simulink model "ABC_model_Group_05"  (R2023a)
settings: Solver=VariableStepAuto  StartTime=0.0  StopTime=10.0  RelTol=1e-3
libraries: sharedutil x6, aerolibutil x2
settings Model: Creator=shivam  LastModifiedBy=shivam

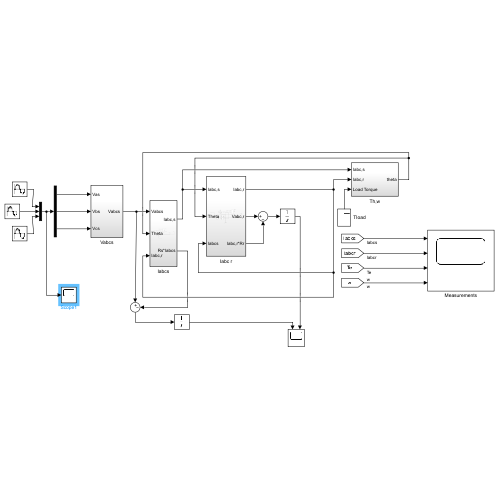
[thumbnail: Simulink's stored preview of the top-level diagram]
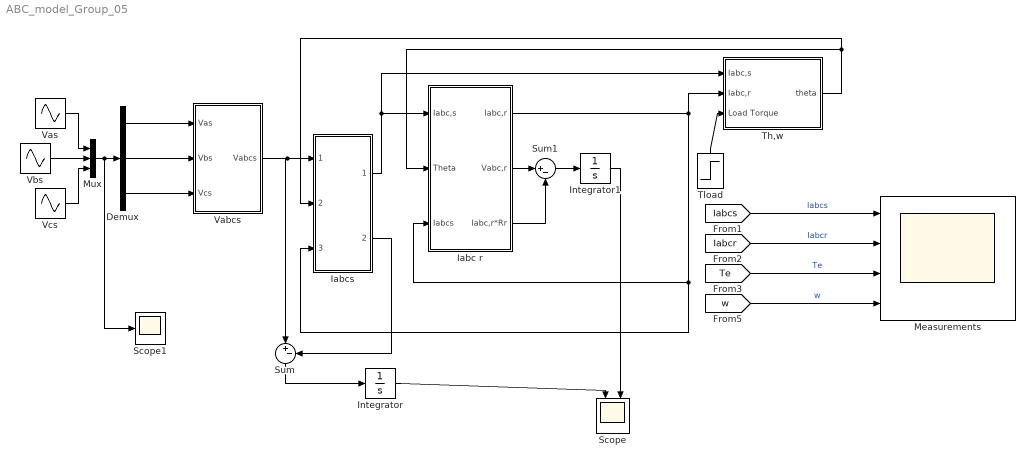
== system ABC_model_Group_05 ==
  Demux : Demux  Outputs=3
  Iabc r : Subsystem
  Iabcs : Subsystem
  Integrator : Integrator
  Integrator1 : Integrator
  "Measurements " : Scope  NumInputPorts=4
  Mux : Mux  Inputs=3
  Scope : Scope  NumInputPorts=2
  Scope1 : Scope
  Sum : Sum  Inputs=|+-
  Sum1 : Sum  Inputs=|+-
  Th,w : Subsystem
  Tload : Step  After=200.106  SampleTime=0
  Vabcs : Subsystem
  Vas : Sin  Amplitude=(460*sqrt(2))/sqrt(3)  Frequency=2*pi*60  Phase=(2*pi)/3  SampleTime=50e-6
  Vbs : Sin  Amplitude=(460*sqrt(2))/sqrt(3)  Frequency=2*pi*60  SampleTime=50e-6
  Vcs : Sin  Amplitude=(460*sqrt(2))/sqrt(3)  Frequency=2*pi*60  Phase=(4*pi)/3  SampleTime=50e-6
  wires:
  Vcs/1 -> Mux/3
  Vas/1 -> Mux/1
  Vbs/1 -> Mux/2
  Demux/3 -> Vabcs/3(Vcs)
  Demux/2 -> Vabcs/2(Vbs)
  Demux/1 -> Vabcs/1(Vas)
  Mux/1 -> Scope1/1, Demux/1
  Tload/1 -> Th,w/3(Load Torque)
  [w] -> "Measurements "/4  "w"
  [Te] -> "Measurements "/3  "Te"
  [Iabcr] -> "Measurements "/2  "Iabcr"
  [Iabcs] -> "Measurements "/1  "Iabcs"
  Vabcs/1("Vabcs ") -> Sum/1, Iabcs/1(Vabcs)
  Iabcs/2(Rs*Iabcs) -> Sum/2
  Sum/1 -> Integrator/1
  Integrator/1 -> Scope/1
  Th,w/1(theta) -> Iabcs/2(Theta), Iabc r/2(Theta)
  Iabcs/1(Iabc,s) -> Iabc r/1(Iabc,s), Th,w/1(Iabc,s)
  Iabc r/1(Iabc,r) -> Th,w/2(Iabc,r), Iabcs/3(Iabc,r), Iabc r/3(Iabcs)
  Iabc r/2(Vabc,r) -> Sum1/1
  Iabc r/3(Iabc,r*Rr) -> Sum1/2
  Sum1/1 -> Integrator1/1
  Integrator1/1 -> Scope/2

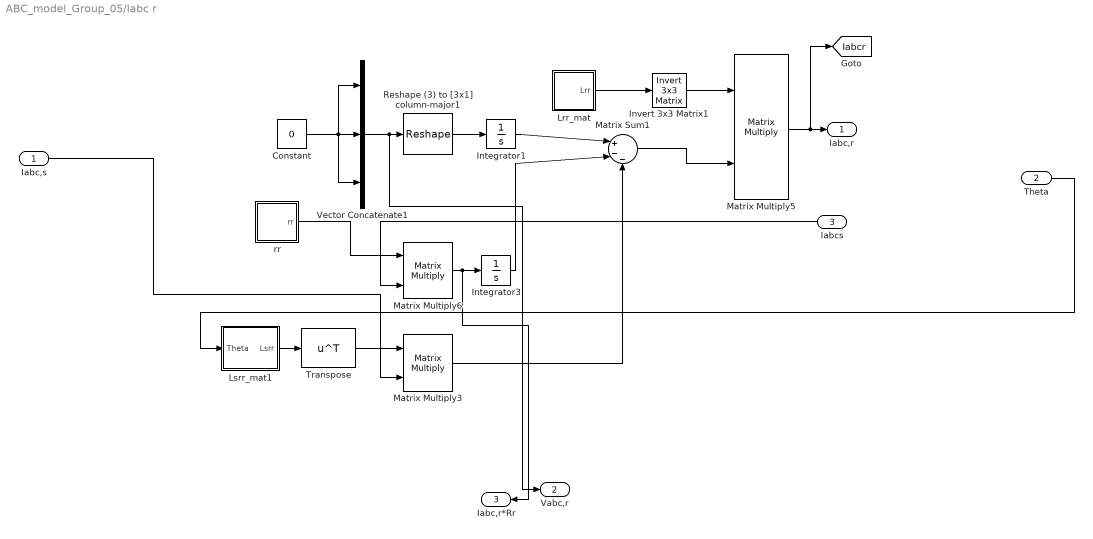
== system ABC_model_Group_05/Iabc r ==
  Iabc,s : Inport
  Theta : Inport  Port=2
  Iabcs : Inport  Port=3
  Constant : Constant  Value=0
  Integrator1 : Integrator
  Integrator3 : Integrator
  Invert 3x3 Matrix1 : aerolibutil/Invert  3x3 Matrix
  Lrr_mat : Subsystem
  Lsrr_mat1 : Subsystem
  Matrix Sum1 : Sum  Inputs=|+--
  Matrix Multiply3 : Product  Multiplication=Matrix(*)
  Matrix Multiply5 : Product  Multiplication=Matrix(*)
  Matrix Multiply6 : Product  Multiplication=Matrix(*)
  Reshape (3) to [3x1] column-major1 : Reshape  OutputDimensionality=Customize  OutputDimensions=[3,1]
  Transpose : Math  Operator=transpose
  Vector Concatenate1 : Concatenate  NumInputs=3
  rr : Subsystem
  Iabc,r : Outport
  Vabc,r : Outport  Port=2
  Iabc,r*Rr : Outport  Port=3
  tag scope: Iabcr=global
  wires:
  Matrix Multiply6/1 -> Iabc,r*Rr/1, Integrator3/1
  Integrator1/1 -> Matrix Sum1/1
  Theta/1 -> Lsrr_mat1/1(Theta)
  Iabc,s/1 -> Matrix Multiply3/2
  Constant/1 -> Vector Concatenate1/3, Vector Concatenate1/1, Vector Concatenate1/2
  Lrr_mat/1(Lrr) -> Invert 3x3 Matrix1/1
  Reshape (3) to [3x1] column-major1/1 -> Integrator1/1
  Vector Concatenate1/1 -> Vabc,r/1, Reshape (3) to [3x1] column-major1/1
  rr/1(rr) -> Matrix Multiply6/1
  Matrix Sum1/1 -> Matrix Multiply5/2
  Matrix Multiply3/1 -> Matrix Sum1/3
  Integrator3/1 -> Matrix Sum1/2
  Invert 3x3 Matrix1/1 -> Matrix Multiply5/1
  Matrix Multiply5/1 -> Iabc,r/1, [Iabcr]
  Iabcs/1 -> Matrix Multiply6/2
  Lsrr_mat1/1(Lsrr) -> Transpose/1
  Transpose/1 -> Matrix Multiply3/1

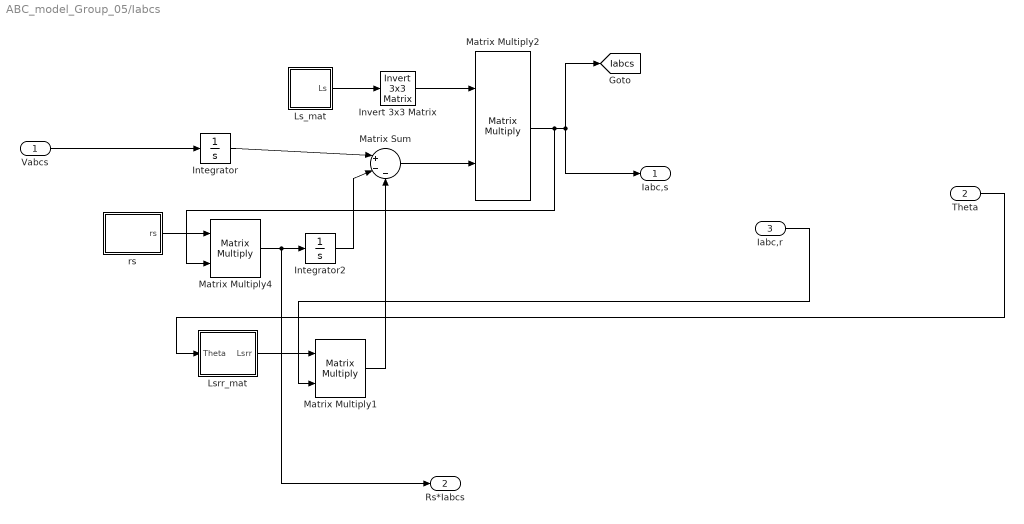
== system ABC_model_Group_05/Iabcs ==
  Vabcs : Inport
  Theta : Inport  Port=2
  Iabc,r : Inport  Port=3
  Integrator : Integrator
  Integrator2 : Integrator
  Invert 3x3 Matrix : aerolibutil/Invert  3x3 Matrix
  Ls_mat : Subsystem
  Lsrr_mat : Subsystem
  Matrix Sum : Sum  Inputs=|+--
  Matrix Multiply1 : Product  Multiplication=Matrix(*)
  Matrix Multiply2 : Product  Multiplication=Matrix(*)
  Matrix Multiply4 : Product  Multiplication=Matrix(*)
  rs : Subsystem
  Iabc,s : Outport
  Rs*Iabcs : Outport  Port=2
  tag scope: Iabcs=global
  wires:
  rs/1(rs) -> Matrix Multiply4/1
  Invert 3x3 Matrix/1 -> Matrix Multiply2/1
  Matrix Multiply4/1 -> Rs*Iabcs/1, Integrator2/1
  Vabcs/1 -> Integrator/1
  Ls_mat/1(Ls) -> Invert 3x3 Matrix/1
  Lsrr_mat/1(Lsrr) -> Matrix Multiply1/1
  Matrix Multiply2/1 -> Iabc,s/1, [Iabcs], Matrix Multiply4/2
  Matrix Multiply1/1 -> Matrix Sum/3
  Integrator2/1 -> Matrix Sum/2
  Matrix Sum/1 -> Matrix Multiply2/2
  Integrator/1 -> Matrix Sum/1
  Theta/1 -> Lsrr_mat/1(Theta)
  Iabc,r/1 -> Matrix Multiply1/2

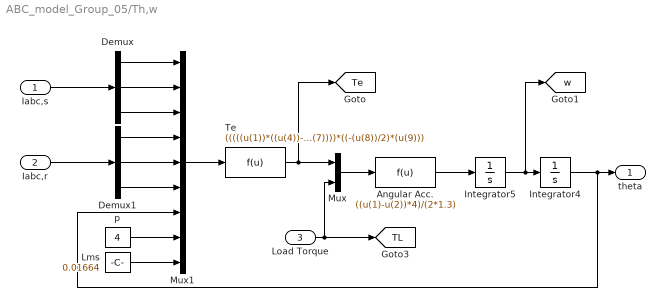
== system ABC_model_Group_05/Th,w ==
  Iabc,s : Inport
  Iabc,r : Inport  Port=2
  Load Torque : Inport  Port=3
  Angular Acc. : Fcn  Expr=((u(1)-u(2))*4)/(2*1.3)
  Demux : Demux  Outputs=3
  Demux1 : Demux  Outputs=3
  Integrator4 : Integrator
  Integrator5 : Integrator
  Lms : Constant  Value=0.01664
  Mux : Mux  Inputs=2
  Mux1 : Mux  Inputs=9
  Te : Fcn  Expr=(((((u(1))*((u(4))-(0.5*(u(5)))-(0.5*(u(6)))))+((u(2))*((u(5))-(0.5*(u(4)))-(0.5*(u(6)))))+((u(3))*((u(6))-(0.5*(u(5)))-(0.5*(u(4))))))*sin(u(7)))+((sqrt(3)/2)*(((u(1))*((u(5))-(u(6))))+((u(2))*((u(6))-(u(4))))+((u(3))*((u(4))-(u(5)))))*cos(u(7))))*((-(u(8))/2)*(u(9)))
  p : Constant  Value=4
  theta : Outport
  tag scope: TL=global, Te=global, w=global
  wires:
  Iabc,s/1 -> Demux/1
  Integrator4/1 -> Mux1/7, theta/1
  Mux/1 -> Angular Acc./1
  Load Torque/1 -> Mux/2, [TL]
  Angular Acc./1 -> Integrator5/1
  Te/1 -> [Te], Mux/1
  Integrator5/1 -> [w], Integrator4/1
  Iabc,r/1 -> Demux1/1
  Mux1/1 -> Te/1
  Demux/1 -> Mux1/1
  Demux/2 -> Mux1/2
  Demux/3 -> Mux1/3
  Demux1/1 -> Mux1/4
  Demux1/2 -> Mux1/5
  Demux1/3 -> Mux1/6
  p/1 -> Mux1/8
  Lms/1 -> Mux1/9

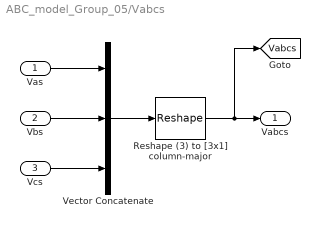
== system ABC_model_Group_05/Vabcs ==
  Vas : Inport
  Vbs : Inport  Port=2
  Vcs : Inport  Port=3
  Reshape (3) to [3x1] column-major : Reshape  OutputDimensionality=Customize  OutputDimensions=[3,1]
  Vector Concatenate : Concatenate  NumInputs=3
  "Vabcs " : Outport
  tag scope: Vabcs=global
  wires:
  Vector Concatenate/1 -> Reshape (3) to [3x1] column-major/1
  Reshape (3) to [3x1] column-major/1 -> [Vabcs], "Vabcs "/1
  Vbs/1 -> Vector Concatenate/2
  Vcs/1 -> Vector Concatenate/3
  Vas/1 -> Vector Concatenate/1

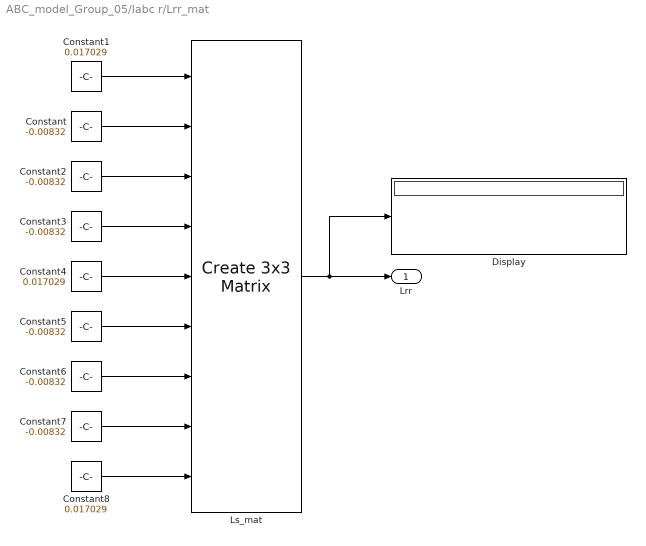
== system ABC_model_Group_05/Iabc r/Lrr_mat ==
  Constant{,2..3,5..7} (6 alike) : Constant  Value=-0.00832
  Constant1 : Constant  Value=0.017029
  Constant4 : Constant  Value=0.017029
  Constant8 : Constant  Value=0.017029
  Display : Display
  Ls_mat : sharedutil/Create 3x3 Matrix  aMode=aMode
      settings: LibrarySourceBlock=aerolibutil/Create 3x3 Matrix
  Lrr : Outport
  wires:
  Constant4/1 -> Ls_mat/5
  Constant5/1 -> Ls_mat/6
  Constant/1 -> Ls_mat/2
  Constant3/1 -> Ls_mat/4
  Constant1/1 -> Ls_mat/1
  Constant2/1 -> Ls_mat/3
  Constant6/1 -> Ls_mat/7
  Constant7/1 -> Ls_mat/8
  Constant8/1 -> Ls_mat/9
  Ls_mat/1 -> Display/1, Lrr/1

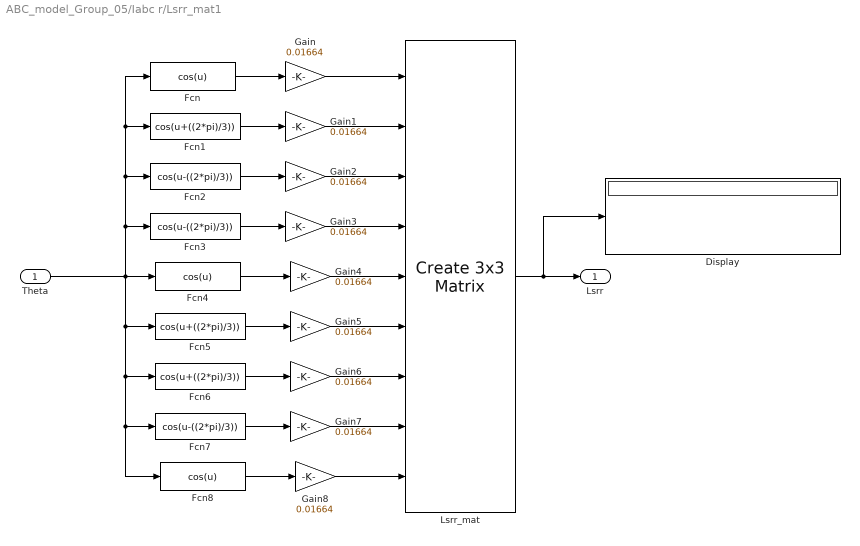
== system ABC_model_Group_05/Iabc r/Lsrr_mat1 ==
  Theta : Inport
  Display : Display
  Fcn : Fcn  Expr=cos(u)
  Fcn1 : Fcn  Expr=cos(u+((2*pi)/3))
  Fcn2 : Fcn  Expr=cos(u-((2*pi)/3))
  Fcn3 : Fcn  Expr=cos(u-((2*pi)/3))
  Fcn4 : Fcn  Expr=cos(u)
  Fcn5 : Fcn  Expr=cos(u+((2*pi)/3))
  Fcn6 : Fcn  Expr=cos(u+((2*pi)/3))
  Fcn7 : Fcn  Expr=cos(u-((2*pi)/3))
  Fcn8 : Fcn  Expr=cos(u)
  Gain{,1..8} (9 alike) : Gain  Gain=0.01664
  Lsrr_mat : sharedutil/Create 3x3 Matrix  aMode=aMode
      settings: LibrarySourceBlock=aerolibutil/Create 3x3 Matrix
  Lsrr : Outport
  wires:
  Fcn/1 -> Gain/1
  Fcn1/1 -> Gain1/1
  Fcn2/1 -> Gain2/1
  Gain/1 -> Lsrr_mat/1
  Gain1/1 -> Lsrr_mat/2
  Gain2/1 -> Lsrr_mat/3
  Fcn3/1 -> Gain3/1
  Gain3/1 -> Lsrr_mat/4
  Fcn4/1 -> Gain4/1
  Gain4/1 -> Lsrr_mat/5
  Fcn5/1 -> Gain5/1
  Gain5/1 -> Lsrr_mat/6
  Fcn6/1 -> Gain6/1
  Gain6/1 -> Lsrr_mat/7
  Fcn7/1 -> Gain7/1
  Gain7/1 -> Lsrr_mat/8
  Fcn8/1 -> Gain8/1
  Gain8/1 -> Lsrr_mat/9
  Theta/1 -> Fcn/1, Fcn1/1, Fcn2/1, Fcn3/1, Fcn5/1, Fcn6/1, Fcn8/1, Fcn7/1, Fcn4/1
  Lsrr_mat/1 -> Display/1, Lsrr/1

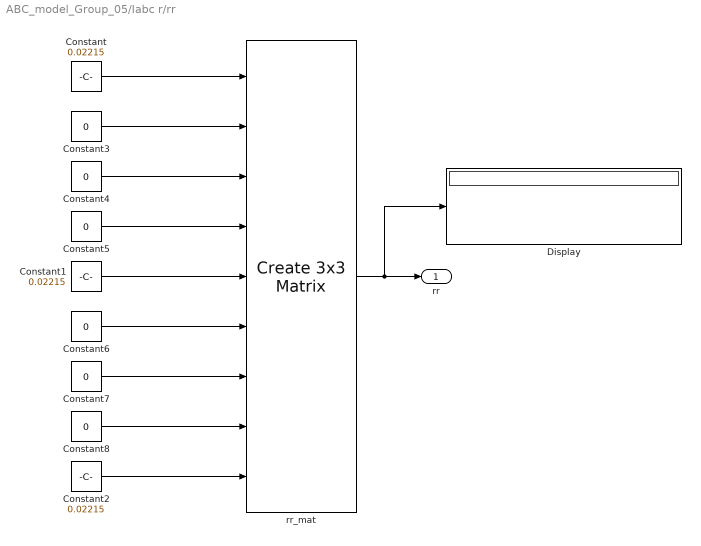
== system ABC_model_Group_05/Iabc r/rr ==
  Constant : Constant  Value=0.02215
  Constant1 : Constant  Value=0.02215
  Constant2 : Constant  Value=0.02215
  Constant{3..8} (6 alike) : Constant  Value=0
  Display : Display
  rr_mat : sharedutil/Create 3x3 Matrix  aMode=aMode
      settings: LibrarySourceBlock=aerolibutil/Create 3x3 Matrix
  rr : Outport
  wires:
  Constant/1 -> rr_mat/1
  Constant3/1 -> rr_mat/2
  Constant4/1 -> rr_mat/3
  Constant5/1 -> rr_mat/4
  Constant1/1 -> rr_mat/5
  Constant6/1 -> rr_mat/6
  Constant7/1 -> rr_mat/7
  Constant8/1 -> rr_mat/8
  Constant2/1 -> rr_mat/9
  rr_mat/1 -> Display/1, rr/1

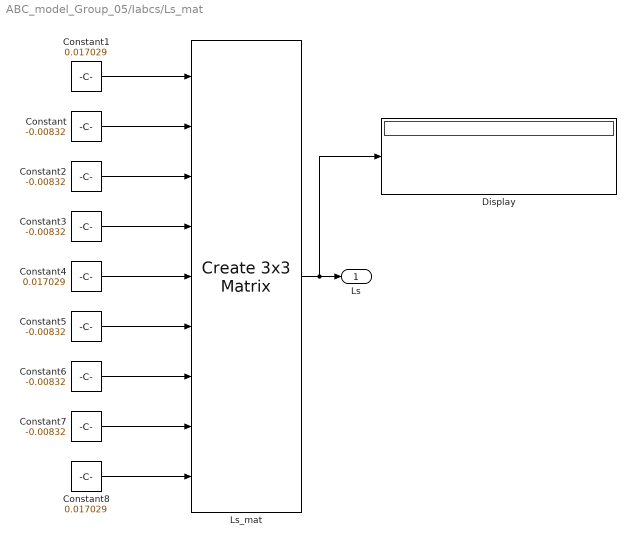
== system ABC_model_Group_05/Iabcs/Ls_mat ==
  Constant{,2..3,5..7} (6 alike) : Constant  Value=-0.00832
  Constant1 : Constant  Value=0.017029
  Constant4 : Constant  Value=0.017029
  Constant8 : Constant  Value=0.017029
  Display : Display
  Ls_mat : sharedutil/Create 3x3 Matrix  aMode=aMode
      settings: LibrarySourceBlock=aerolibutil/Create 3x3 Matrix
  Ls : Outport
  wires:
  Constant4/1 -> Ls_mat/5
  Constant5/1 -> Ls_mat/6
  Constant/1 -> Ls_mat/2
  Constant3/1 -> Ls_mat/4
  Constant1/1 -> Ls_mat/1
  Constant2/1 -> Ls_mat/3
  Constant6/1 -> Ls_mat/7
  Constant7/1 -> Ls_mat/8
  Constant8/1 -> Ls_mat/9
  Ls_mat/1 -> Display/1, Ls/1

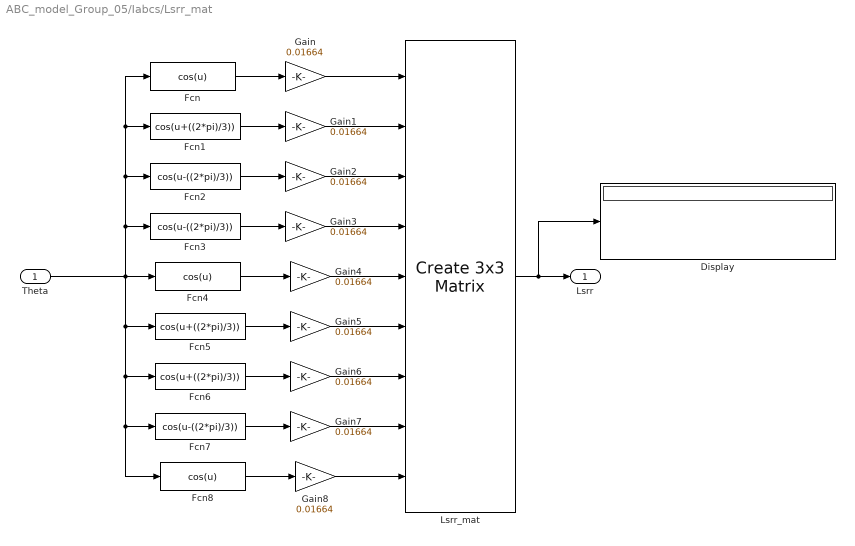
== system ABC_model_Group_05/Iabcs/Lsrr_mat ==
  Theta : Inport
  Display : Display
  Fcn : Fcn  Expr=cos(u)
  Fcn1 : Fcn  Expr=cos(u+((2*pi)/3))
  Fcn2 : Fcn  Expr=cos(u-((2*pi)/3))
  Fcn3 : Fcn  Expr=cos(u-((2*pi)/3))
  Fcn4 : Fcn  Expr=cos(u)
  Fcn5 : Fcn  Expr=cos(u+((2*pi)/3))
  Fcn6 : Fcn  Expr=cos(u+((2*pi)/3))
  Fcn7 : Fcn  Expr=cos(u-((2*pi)/3))
  Fcn8 : Fcn  Expr=cos(u)
  Gain{,1..8} (9 alike) : Gain  Gain=0.01664
  Lsrr_mat : sharedutil/Create 3x3 Matrix  aMode=aMode
      settings: LibrarySourceBlock=aerolibutil/Create 3x3 Matrix
  Lsrr : Outport
  wires:
  Fcn/1 -> Gain/1
  Fcn1/1 -> Gain1/1
  Fcn2/1 -> Gain2/1
  Gain/1 -> Lsrr_mat/1
  Gain1/1 -> Lsrr_mat/2
  Gain2/1 -> Lsrr_mat/3
  Fcn3/1 -> Gain3/1
  Gain3/1 -> Lsrr_mat/4
  Fcn4/1 -> Gain4/1
  Gain4/1 -> Lsrr_mat/5
  Fcn5/1 -> Gain5/1
  Gain5/1 -> Lsrr_mat/6
  Fcn6/1 -> Gain6/1
  Gain6/1 -> Lsrr_mat/7
  Fcn7/1 -> Gain7/1
  Gain7/1 -> Lsrr_mat/8
  Fcn8/1 -> Gain8/1
  Gain8/1 -> Lsrr_mat/9
  Theta/1 -> Fcn/1, Fcn1/1, Fcn2/1, Fcn3/1, Fcn5/1, Fcn6/1, Fcn8/1, Fcn7/1, Fcn4/1
  Lsrr_mat/1 -> Display/1, Lsrr/1

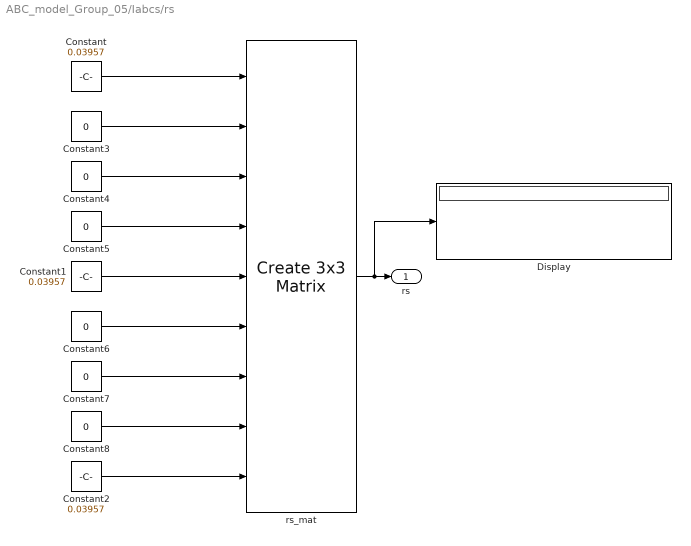
== system ABC_model_Group_05/Iabcs/rs ==
  Constant : Constant  Value=0.03957
  Constant1 : Constant  Value=0.03957
  Constant2 : Constant  Value=0.03957
  Constant{3..8} (6 alike) : Constant  Value=0
  Display : Display
  rs_mat : sharedutil/Create 3x3 Matrix  aMode=aMode
      settings: LibrarySourceBlock=aerolibutil/Create 3x3 Matrix
  rs : Outport
  wires:
  rs_mat/1 -> Display/1, rs/1
  Constant/1 -> rs_mat/1
  Constant3/1 -> rs_mat/2
  Constant4/1 -> rs_mat/3
  Constant5/1 -> rs_mat/4
  Constant1/1 -> rs_mat/5
  Constant6/1 -> rs_mat/6
  Constant7/1 -> rs_mat/7
  Constant8/1 -> rs_mat/8
  Constant2/1 -> rs_mat/9
